simulink model "MdL_iyi"  (R2018a)
settings: Solver=ode4  StartTime=0.0  StopTime=5  FixedStep=0.001  RelTol=1e-3
values from neighbouring files (symbols this model uses):
  A = [0 1;8.04915 -0.09255]    [qiyi.m]
  B = [0;-8.92329]    [qiyi.m]
  C = [1 0;0 1]    [qiyi.m]
  delta_A = [0 0; 1.48068 -0.00318]*state_model    [qiyi.m]
  delta_B = [0;-0.04781]*state_model    [qiyi.m]
  K = place(A,B,P)*inv(C)    [qiyi.m]
  L = N'    [qiyi.m]
settings Model: Creator=80741  LastModifiedBy=80741
settings DataIOCC: LimitDataPoints=on  SaveFormat=Array  SignalLoggingSaveFormat=ModelDataLogs
settings OptimizationCC: InitFltsAndDblsToZero=on  LifeSpan=inf
settings DebuggingCC: SaveWithParameterizedLinksMsg=none  UnderspecifiedInitializationDetection=Classic  MergeDetectMultiDrivingBlocksExec=none  SignalResolutionControl=TryResolveAllWithWarning  SolverPrmCheckMsg=warning  MultiTaskDSMMsg=warning  MultiTaskCondExecSysMsg=none  FcnCallInpInsideContextMsg=warning  SFUnexpectedBacktrackingDiag=warning  SFNoUnconditionalDefaultTransitionDiag=warning  SFExecutionAtInitializationDiag=none
settings HardwareCC: ProdBitPerPointer=32  ProdBitPerSizeT=32  ProdBitPerPtrDiffT=32  ProdLargestAtomicFloat=None  ProdIntDivRoundTo=Undefined  ProdEndianess=Unspecified  ProdWordSize=32  ProdHWDeviceType=32-bit Generic
settings ModelReferenceCC: PropagateSignalLabelsOutOfModel=off
settings CodeAppCC: StateflowObjectComments=on
settings GRTTargetCC: TargetFcnLib=ansi_tfl_tmw.mat  TargetLangStandard=C89/C90 (ANSI)  CombineOutputUpdateFcns=off  GRTInterface=on
settings ConfigComp: CovMetricSettings=dw  CovHtmlReporting=on  CovSaveCumulativeToWorkspaceVar=on  CovSaveSingleToWorkspaceVar=on  CovExternalEMLEnable=off

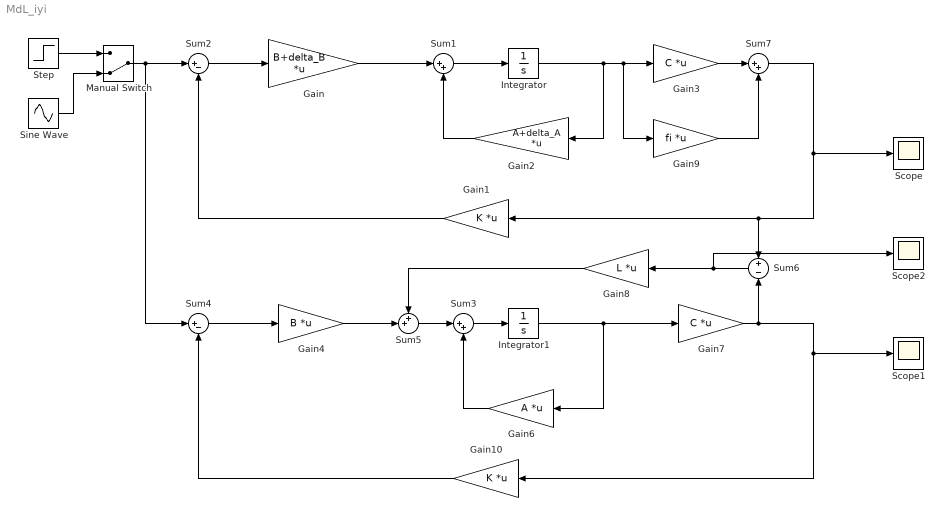
== system MdL_iyi ==
  Gain : Gain  Gain=B+delta_B  Multiplication=Matrix(K*u)
  Gain1 : Gain  Gain=K  Multiplication=Matrix(K*u)
  Gain10 : Gain  Gain=K  Multiplication=Matrix(K*u)
  Gain2 : Gain  Gain=A+delta_A  Multiplication=Matrix(K*u)
  Gain3 : Gain  Gain=C  Multiplication=Matrix(K*u)
  Gain4 : Gain  Gain=B  Multiplication=Matrix(K*u)
  Gain6 : Gain  Gain=A  Multiplication=Matrix(K*u)
  Gain7 : Gain  Gain=C  Multiplication=Matrix(K*u)
  Gain8 : Gain  Gain=L  Multiplication=Matrix(K*u)
  Gain9 : Gain  Gain=fi  Multiplication=Matrix(K*u)
  Integrator : Integrator  InitialCondition=[2;1]
  Integrator1 : Integrator
  Manual Switch : ManualSwitch  CurrentSetting=0
  Scope : Scope
  Scope1 : Scope
  Scope2 : Scope
  Sine Wave : Sin  SampleTime=0
  Step : Step  Time=0  SampleTime=0
  Sum1 : Sum  Inputs=|++
  Sum2 : Sum  Inputs=|+-
  Sum3 : Sum  Inputs=|++
  Sum4 : Sum  Inputs=|+-
  Sum5 : Sum  Inputs=++|
  Sum6 : Sum  Inputs=+-
  Sum7 : Sum  Inputs=|++
  wires:
  Manual Switch/1 -> Sum2/1, Sum4/1
  Gain/1 -> Sum1/1
  Sum1/1 -> Integrator/1
  Integrator/1 -> Gain2/1, Gain3/1, Gain9/1
  Sum2/1 -> Gain/1
  Sum3/1 -> Integrator1/1
  Integrator1/1 -> Gain7/1, Gain6/1
  Gain6/1 -> Sum3/2
  Sum4/1 -> Gain4/1
  Sum5/1 -> Sum3/1
  Sum7/1 -> Scope/1, Sum6/1, Gain1/1
  Step/1 -> Manual Switch/1
  Sine Wave/1 -> Manual Switch/2
  Gain2/1 -> Sum1/2
  Gain3/1 -> Sum7/1
  Gain4/1 -> Sum5/2
  Gain8/1 -> Sum5/1
  Gain1/1 -> Sum2/2
  Gain10/1 -> Sum4/2
  Sum6/1 -> Scope2/1, Gain8/1
  Gain7/1 -> Sum6/2, Scope1/1, Gain10/1
  Gain9/1 -> Sum7/2
